simulink model "sim_tvt_2025_pos_ctrl"  (R2020a)
settings: Solver=ode4  StartTime=0.0  StopTime=30.0  FixedStep=0.01  RelTol=1e-3
values from neighbouring files (symbols this model uses):
  alfa = 0.02    [init_tvt_2025_pos_ctrl.m]
  alfa_theta = 20    [init_tvt_2025_pos_ctrl.m]
  alfa_theta_obs = 100    [init_tvt_2025_pos_ctrl.m]
  c0 = 0.1    [init_tvt_2025_pos_ctrl.m]
  c1_diff_sigma_bar_v = diag([25; 30; 20])    [init_tvt_2025_pos_ctrl.m]
  c1v = diag([5.8; 6.5; 6.5])    [init_tvt_2025_pos_ctrl.m]
  c2_diff_sigma_bar_v = diag([50; 50; 10])    [init_tvt_2025_pos_ctrl.m]
  c2v = diag([5.8; 6.5; 6.5])    [init_tvt_2025_pos_ctrl.m]
  c3_diff_sigma_bar_v = diag([15; 15; 10])    [init_tvt_2025_pos_ctrl.m]
  c3v = diag([4.8; 6.4; 6.0])    [init_tvt_2025_pos_ctrl.m]
  delta_p_i_0 = zeros(3, NF)    [init_tvt_2025_pos_ctrl.m]
  delta_v_i_0 = zeros(3, NF)    [init_tvt_2025_pos_ctrl.m]
  dp_aa_t = 0.2 * ones(3, 5) + ( 1.0 - 0.2 ) * rand(3, 5)    [init_tvt_2025_pos_ctrl.m]
  dp_ff_t = [ 0.4 * ones(1, 5) + ( 1.0 - 0.4 ) * rand(1, 5);                      0.4 * ones(1, 5) + ( 1.0 - 0.4 ) * rand(1, 5);                      0.2 * ones(1, 5) + ( 0.6 - 0.2 ) * rand(1, 5) ]    [init_tvt_2025_pos_ctrl.m]
  dp_phi_t = ( - pi / 2 ) * ones(3, 5) + ( pi / 2 - ( - pi / 2 ) ) * rand(3, 5)    [init_tvt_2025_pos_ctrl.m]
  eps0 = [0.05; 0.01; 0.01]    [init_tvt_2025_pos_ctrl.m]
  eta_ld_hat_init = zeros(3,NF)    [init_tvt_2025_pos_ctrl.m]
  etai_0 = zeros(3,5)    [init_tvt_2025_pos_ctrl.m]
  gamma0 = diag([1, 1, 1])    [init_tvt_2025_pos_ctrl.m]
  k_phi = diag([10, 10, 10])    [init_tvt_2025_pos_ctrl.m]
  k_theta = diag([5, 5, 5])    [init_tvt_2025_pos_ctrl.m]
  kai0 = [15; 10; 10]    [init_tvt_2025_pos_ctrl.m]
  kai_1_t = 0.02    [init_tvt_2025_pos_ctrl.m]
  kai_3_t = 0.1    [init_tvt_2025_pos_ctrl.m]
  ksi_ld_hat_init = zeros(3,NF)    [init_tvt_2025_pos_ctrl.m]
  ksii_0 = zeros(3,5)    [init_tvt_2025_pos_ctrl.m]
  l1v = diag([20; 20; 20])    [init_tvt_2025_pos_ctrl.m]
  l2v = diag([30; 30; 30])    [init_tvt_2025_pos_ctrl.m]
  lam0 = [15; 10; 10]    [init_tvt_2025_pos_ctrl.m]
  lam1 = diag([5,5,5])    [init_tvt_2025_pos_ctrl.m]
  lam2 = diag([5,5,5])    [init_tvt_2025_pos_ctrl.m]
  lam3 = diag([5,5,5])    [init_tvt_2025_pos_ctrl.m]
  lam4 = diag([5,5,5])    [init_tvt_2025_pos_ctrl.m]
  Lamd_diff_sigma_bar_v = 0.5    [init_tvt_2025_pos_ctrl.m]
  mass_i = zeros(1,NF)    [init_tvt_2025_pos_ctrl.m]
  Mii = diag([1;0;0;0;1])    [init_tvt_2025_pos_ctrl.m]
  pos0 = zeros(3, 1)    [init_tvt_2025_pos_ctrl.m]
  pos_bar_init = zeros(3,NF)    [init_tvt_2025_pos_ctrl.m]
  PZ0 = P0(3)    [init_tvt_2025_pos_ctrl.m]
  PZ1 = 10    [init_tvt_2025_pos_ctrl.m]
  Qci_init = repmat([1;0;0;0],1,NF)    [init_tvt_2025_pos_ctrl.m]
  R0 = 4    [init_tvt_2025_pos_ctrl.m]
  R1 = 8    [init_tvt_2025_pos_ctrl.m]
  Rx2 = 10    [init_tvt_2025_pos_ctrl.m]
  Ry2 = 6    [init_tvt_2025_pos_ctrl.m]
  Rz2 = 4    [init_tvt_2025_pos_ctrl.m]
  T0 = 0    [init_tvt_2025_pos_ctrl.m]
  T1 = tseq1    (= 10)    [init_tvt_2025_pos_ctrl.m]
  T12 = tseq1 + tseq12    (= 20)    [init_tvt_2025_pos_ctrl.m]
  T2 = tseq1 + tseq12 + tseq2    (= 30)    [init_tvt_2025_pos_ctrl.m]
  theta0 = ( 2 / 5 ) * pi    (= 1.25663706144)    [init_tvt_2025_pos_ctrl.m]
  vel0 = zeros(3, 1)    [init_tvt_2025_pos_ctrl.m]
  vel_bar_init = zeros(3,NF)    [init_tvt_2025_pos_ctrl.m]
  Wij = [0,0,1,0,0;              0,0,1,1,0;              1,0,0,0,1;              0,1,1,0,0;              0,0,1,0,0]    [init_tvt_2025_pos_ctrl.m]
  X1 = 8    [init_tvt_2025_pos_ctrl.m]
  X2 = 2    [init_tvt_2025_pos_ctrl.m]
  X3 = 3    [init_tvt_2025_pos_ctrl.m]
  Y1 = 10    [init_tvt_2025_pos_ctrl.m]
  Y2 = 2    [init_tvt_2025_pos_ctrl.m]
  Y3 = 4    [init_tvt_2025_pos_ctrl.m]
  Z1 = 4    [init_tvt_2025_pos_ctrl.m]
  Z2 = -6    [init_tvt_2025_pos_ctrl.m]
  Z3 = 2    [init_tvt_2025_pos_ctrl.m]
  zeta_diff_sigma_bar_v = 0.08    [init_tvt_2025_pos_ctrl.m]
undefined symbols (not defined in the file or in its folder): cal_frac_squ, p_alfav1, p_alfav2, p_gamma1_pos, p_gamma1_vel, p_gamma2_pos, p_gamma2_vel, q_alfav1, q_alfav2, q_gamma1_pos, q_gamma1_vel, q_gamma2_pos, q_gamma2_vel
(part 3 of 5)

== matlab function sim_tvt_2025_pos_ctrl/cal differentiator d_sigma_bar_v_hat agent 3/cal sig3 ==
  data: x input; z output; y input
function z = fcn(x, y)
z = x(:) .* sign(y(:));

== matlab function sim_tvt_2025_pos_ctrl/cal differentiator d_sigma_bar_v_hat agent 3/cal sig4 ==
  data: x input; z output; y input
function z = fcn(x, y)
z = x(:) .* sign(y(:));

== matlab function sim_tvt_2025_pos_ctrl/cal differentiator d_sigma_bar_v_hat agent 3/cal sig5 ==
  data: x input; z output; y input
function z = fcn(x, y)
z = x(:) .* sign(y(:));

== matlab function sim_tvt_2025_pos_ctrl/cal pos_bar_i agent 1 ==
  data: ksi_i_vec input; phi_vec input; pos_bar_1 output
function pos_bar_1 = fcn(ksi_i_vec, phi_vec)
%%%% 计算辅助位置向量
iiuav = 1;
pos_bar_1 = ksi_i_vec(:,iiuav) - phi_vec(:,iiuav);

== matlab function sim_tvt_2025_pos_ctrl/cal pos_bar_i agent 2 ==
  data: ksi_i_vec input; phi_vec input; pos_bar_2 output
function pos_bar_2 = fcn(ksi_i_vec, phi_vec)
%%%% 计算辅助位置向量
iiuav = 2;
pos_bar_2 = ksi_i_vec(:,iiuav) - phi_vec(:,iiuav);

== matlab function sim_tvt_2025_pos_ctrl/cal differentiator d_sigma_bar_v_hat agent 3/choose sigma_bar_v ==
  data: x input; y output
function y = fcn(x)
iiuav = 3;
y = x(:,iiuav);

== matlab function sim_tvt_2025_pos_ctrl/Phi_sec_sigma_i agent 1 ==
  data: sigma_i_vec input; Phi_sec_sigma_1 output
function Phi_sec_sigma_1 = fcn(sigma_i_vec)
%%%% 跟随者期望速度分布式观测器
iiuav = 1;
Phi_sec_sigma_1 = diag( [ sech( sigma_i_vec(1,iiuav) ) ^ 2, ...
                                                sech( sigma_i_vec(2,iiuav) ) ^ 2, ...
                                                sech( sigma_i_vec(3,iiuav) ) ^ 2 ] );

== matlab function sim_tvt_2025_pos_ctrl/cal differentiator d_sigma_bar_v_hat agent 3/trans to column20 ==
  data: x input; y output
function y = fcn(x)
y = x(:);

== matlab function sim_tvt_2025_pos_ctrl/cal differentiator d_sigma_bar_v_hat agent 3/trans to column21 ==
  data: x input; y output
function y = fcn(x)
y = x(:);

== matlab function sim_tvt_2025_pos_ctrl/cal differentiator d_sigma_bar_v_hat agent 3/trans to column22 ==
  data: x input; y output
function y = fcn(x)
y = x(:);

== matlab function sim_tvt_2025_pos_ctrl/cal differentiator d_sigma_bar_v_hat agent 3/trans to column23 ==
  data: x input; y output
function y = fcn(x)
y = x(:);

== matlab function sim_tvt_2025_pos_ctrl/cal differentiator d_sigma_bar_v_hat agent 3/trans to column24 ==
  data: x input; y output
function y = fcn(x)
y = x(:);

== matlab function sim_tvt_2025_pos_ctrl/cal differentiator d_sigma_bar_v_hat agent 3/trans to column25 ==
  data: x input; y output
function y = fcn(x)
y = x(:);

== matlab function sim_tvt_2025_pos_ctrl/cal differentiator d_sigma_bar_v_hat agent 4/cal differentiator ==
  data: c1 input; d_sigma_bar_v_hat output; d_dsigma_bar_v_hat output; d_d2sigma_bar_v_hat output; c2 input; c3 input; chi_t input; sigma_bar_v_sig_1 input; sigma_bar_v_sig_2 input; sigma_bar_v_sig_3 input; sigma_bar_v_sig_4 input; sigma_bar_v_sig_5 input; sigma_bar_v_sig_6 input; d_sigma_bar_v_hat input; d2_sigma_bar_v_hat input
function [d_sigma_bar_v_hat, d_dsigma_bar_v_hat, d_d2sigma_bar_v_hat] = fcn(c1, c2, c3, chi_t, sigma_bar_v_sig_1, sigma_bar_v_sig_2, sigma_bar_v_sig_3, ...
                                                                                                                                                sigma_bar_v_sig_4, sigma_bar_v_sig_5, sigma_bar_v_sig_6, d_sigma_bar_v_hat, d2_sigma_bar_v_hat)
d_d2sigma_bar_v_hat = -chi_t .* c1 * sigma_bar_v_sig_1(:) - (1 - chi_t) .* c1 * sigma_bar_v_sig_2(:);
d_dsigma_bar_v_hat = -chi_t .* c2 * sigma_bar_v_sig_3(:) - (1 - chi_t) .* c2 * sigma_bar_v_sig_4(:) + d2_sigma_bar_v_hat(:);
d_sigma_bar_v_hat = -chi_t .* c3 * sigma_bar_v_sig_5(:) - (1 - chi_t) .* c3 * sigma_bar_v_sig_6(:) + d_sigma_bar_v_hat(:);

== matlab function sim_tvt_2025_pos_ctrl/cal differentiator d_sigma_bar_v_hat agent 4/cal sig ==
  data: x input; z output; y input
function z = fcn(x, y)
z = x(:) .* sign(y(:));

== matlab function sim_tvt_2025_pos_ctrl/Phi_sec_sigma_i agent 2 ==
  data: sigma_i_vec input; Phi_sec_sigma_2 output
function Phi_sec_sigma_2 = fcn(sigma_i_vec)
%%%% 跟随者期望速度分布式观测器
iiuav = 2;
Phi_sec_sigma_2 = diag( [ sech( sigma_i_vec(1,iiuav) ) ^ 2, ...
                                                sech( sigma_i_vec(2,iiuav) ) ^ 2, ...
                                                sech( sigma_i_vec(3,iiuav) ) ^ 2 ] );

== matlab function sim_tvt_2025_pos_ctrl/cal differentiator d_sigma_bar_v_hat agent 4/cal sig1 ==
  data: x input; z output; y input
function z = fcn(x, y)
z = x(:) .* sign(y(:));

== matlab function sim_tvt_2025_pos_ctrl/cal differentiator d_sigma_bar_v_hat agent 4/cal sig2 ==
  data: x input; z output; y input
function z = fcn(x, y)
z = x(:) .* sign(y(:));

== matlab function sim_tvt_2025_pos_ctrl/cal differentiator d_sigma_bar_v_hat agent 4/cal sig3 ==
  data: x input; z output; y input
function z = fcn(x, y)
z = x(:) .* sign(y(:));

== matlab function sim_tvt_2025_pos_ctrl/cal differentiator d_sigma_bar_v_hat agent 4/cal sig4 ==
  data: x input; z output; y input
function z = fcn(x, y)
z = x(:) .* sign(y(:));

== matlab function sim_tvt_2025_pos_ctrl/cal differentiator d_sigma_bar_v_hat agent 4/cal sig5 ==
  data: x input; z output; y input
function z = fcn(x, y)
z = x(:) .* sign(y(:));

== matlab function sim_tvt_2025_pos_ctrl/cal differentiator d_sigma_bar_v_hat agent 4/choose sigma_bar_v ==
  data: x input; y output
function y = fcn(x)
iiuav = 4;
y = x(:,iiuav);

== matlab function sim_tvt_2025_pos_ctrl/cal differentiator d_sigma_bar_v_hat agent 4/trans to column20 ==
  data: x input; y output
function y = fcn(x)
y = x(:);

== matlab function sim_tvt_2025_pos_ctrl/cal differentiator d_sigma_bar_v_hat agent 4/trans to column21 ==
  data: x input; y output
function y = fcn(x)
y = x(:);

== matlab function sim_tvt_2025_pos_ctrl/cal differentiator d_sigma_bar_v_hat agent 4/trans to column22 ==
  data: x input; y output
function y = fcn(x)
y = x(:);

== matlab function sim_tvt_2025_pos_ctrl/Phi_sec_sigma_i agent 3 ==
  data: sigma_i_vec input; Phi_sec_sigma_3 output
function Phi_sec_sigma_3 = fcn(sigma_i_vec)
%%%% 跟随者期望速度分布式观测器
iiuav = 3;
Phi_sec_sigma_3 = diag( [ sech( sigma_i_vec(1,iiuav) ) ^ 2, ...
                                                sech( sigma_i_vec(2,iiuav) ) ^ 2, ...
                                                sech( sigma_i_vec(3,iiuav) ) ^ 2 ] );

== matlab function sim_tvt_2025_pos_ctrl/cal differentiator d_sigma_bar_v_hat agent 4/trans to column23 ==
  data: x input; y output
function y = fcn(x)
y = x(:);

== matlab function sim_tvt_2025_pos_ctrl/cal Rci from ui ==
  data: Rci output; mi_vec input; ui_vec input
function Rci = fcn(mi_vec, ui_vec)
Rci = zeros(3,3,5);
for iiuav = 1:5
    Rci(:,:,iiuav) = cal_Rc_with_u(mi_vec(iiuav), ui_vec(:,iiuav));
end

end

== matlab function sim_tvt_2025_pos_ctrl/cal differentiator d_sigma_bar_v_hat agent 4/trans to column24 ==
  data: x input; y output
function y = fcn(x)
y = x(:);

== matlab function sim_tvt_2025_pos_ctrl/cal differentiator d_sigma_bar_v_hat agent 4/trans to column25 ==
  data: x input; y output
function y = fcn(x)
y = x(:);

== matlab function sim_tvt_2025_pos_ctrl/cal differentiator d_sigma_bar_v_hat agent 5/cal differentiator ==
  data: c1 input; d_sigma_bar_v_hat output; d_dsigma_bar_v_hat output; d_d2sigma_bar_v_hat output; c2 input; c3 input; chi_t input; sigma_bar_v_sig_1 input; sigma_bar_v_sig_2 input; sigma_bar_v_sig_3 input; sigma_bar_v_sig_4 input; sigma_bar_v_sig_5 input; sigma_bar_v_sig_6 input; d_sigma_bar_v_hat input; d2_sigma_bar_v_hat input
function [d_sigma_bar_v_hat, d_dsigma_bar_v_hat, d_d2sigma_bar_v_hat] = fcn(c1, c2, c3, chi_t, sigma_bar_v_sig_1, sigma_bar_v_sig_2, sigma_bar_v_sig_3, ...
                                                                                                                                                sigma_bar_v_sig_4, sigma_bar_v_sig_5, sigma_bar_v_sig_6, d_sigma_bar_v_hat, d2_sigma_bar_v_hat)
d_d2sigma_bar_v_hat = -chi_t .* c1 * sigma_bar_v_sig_1(:) - (1 - chi_t) .* c1 * sigma_bar_v_sig_2(:);
d_dsigma_bar_v_hat = -chi_t .* c2 * sigma_bar_v_sig_3(:) - (1 - chi_t) .* c2 * sigma_bar_v_sig_4(:) + d2_sigma_bar_v_hat(:);
d_sigma_bar_v_hat = -chi_t .* c3 * sigma_bar_v_sig_5(:) - (1 - chi_t) .* c3 * sigma_bar_v_sig_6(:) + d_sigma_bar_v_hat(:);

== matlab function sim_tvt_2025_pos_ctrl/cal differentiator d_sigma_bar_v_hat agent 5/cal sig ==
  data: x input; z output; y input
function z = fcn(x, y)
z = x(:) .* sign(y(:));

== matlab function sim_tvt_2025_pos_ctrl/cal differentiator d_sigma_bar_v_hat agent 5/cal sig1 ==
  data: x input; z output; y input
function z = fcn(x, y)
z = x(:) .* sign(y(:));

== matlab function sim_tvt_2025_pos_ctrl/cal differentiator d_sigma_bar_v_hat agent 5/cal sig2 ==
  data: x input; z output; y input
function z = fcn(x, y)
z = x(:) .* sign(y(:));

== matlab function sim_tvt_2025_pos_ctrl/Phi_sec_sigma_i agent 4 ==
  data: sigma_i_vec input; Phi_sec_sigma_4 output
function Phi_sec_sigma_4 = fcn(sigma_i_vec)
%%%% 跟随者期望速度分布式观测器
iiuav = 4;
Phi_sec_sigma_4 = diag( [ sech( sigma_i_vec(1,iiuav) ) ^ 2, ...
                                                sech( sigma_i_vec(2,iiuav) ) ^ 2, ...
                                                sech( sigma_i_vec(3,iiuav) ) ^ 2 ] );

== matlab function sim_tvt_2025_pos_ctrl/cal differentiator d_sigma_bar_v_hat agent 5/cal sig3 ==
  data: x input; z output; y input
function z = fcn(x, y)
z = x(:) .* sign(y(:));

== matlab function sim_tvt_2025_pos_ctrl/cal differentiator d_sigma_bar_v_hat agent 5/cal sig4 ==
  data: x input; z output; y input
function z = fcn(x, y)
z = x(:) .* sign(y(:));

== matlab function sim_tvt_2025_pos_ctrl/cal differentiator d_sigma_bar_v_hat agent 5/cal sig5 ==
  data: x input; z output; y input
function z = fcn(x, y)
z = x(:) .* sign(y(:));

== matlab function sim_tvt_2025_pos_ctrl/cal differentiator d_sigma_bar_v_hat agent 5/choose sigma_bar_v ==
  data: x input; y output
function y = fcn(x)
iiuav = 5;
y = x(:,iiuav);

== matlab function sim_tvt_2025_pos_ctrl/cal differentiator d_sigma_bar_v_hat agent 5/trans to column20 ==
  data: x input; y output
function y = fcn(x)
y = x(:);

== matlab function sim_tvt_2025_pos_ctrl/cal differentiator d_sigma_bar_v_hat agent 5/trans to column21 ==
  data: x input; y output
function y = fcn(x)
y = x(:);

== matlab function sim_tvt_2025_pos_ctrl/cal differentiator d_sigma_bar_v_hat agent 5/trans to column22 ==
  data: x input; y output
function y = fcn(x)
y = x(:);

== matlab function sim_tvt_2025_pos_ctrl/cal differentiator d_sigma_bar_v_hat agent 5/trans to column23 ==
  data: x input; y output
function y = fcn(x)
y = x(:);

== matlab function sim_tvt_2025_pos_ctrl/cal differentiator d_sigma_bar_v_hat agent 5/trans to column24 ==
  data: x input; y output
function y = fcn(x)
y = x(:);

== matlab function sim_tvt_2025_pos_ctrl/Phi_sec_sigma_i agent 5 ==
  data: sigma_i_vec input; Phi_sec_sigma_5 output
function Phi_sec_sigma_5 = fcn(sigma_i_vec)
%%%% 跟随者期望速度分布式观测器
iiuav = 5;
Phi_sec_sigma_5 = diag( [ sech( sigma_i_vec(1,iiuav) ) ^ 2, ...
                                                sech( sigma_i_vec(2,iiuav) ) ^ 2, ...
                                                sech( sigma_i_vec(3,iiuav) ) ^ 2 ] );

== matlab function sim_tvt_2025_pos_ctrl/cal differentiator d_sigma_bar_v_hat agent 5/trans to column25 ==
  data: x input; y output
function y = fcn(x)
y = x(:);

== matlab function sim_tvt_2025_pos_ctrl/combine d_sigma_bar_v_est ==
  data: d_sigma_bar_v_est_1 input; d_sigma_bar_v_est_2 input; d_sigma_bar_v_est_3 input; d_sigma_bar_v_est_4 input; d_sigma_bar_v_est_5 input; d_sigma_bar_v_vec output
function d_sigma_bar_v_vec  = fcn(d_sigma_bar_v_est_1, d_sigma_bar_v_est_2, d_sigma_bar_v_est_3, d_sigma_bar_v_est_4, d_sigma_bar_v_est_5)
%%%% 合并用微分器求得的虚拟速度控制量导数
d_sigma_bar_v_vec = [d_sigma_bar_v_est_1(:), d_sigma_bar_v_est_2(:), d_sigma_bar_v_est_3(:), d_sigma_bar_v_est_4(:), d_sigma_bar_v_est_5(:)];

== matlab function sim_tvt_2025_pos_ctrl/cal abs 21 ==
  data: x input; y output
function y = fcn(x)
y = abs(x(:));

== matlab function sim_tvt_2025_pos_ctrl/cal abs 22 ==
  data: x input; y output
function y = fcn(x)
y = abs(x(:));

== matlab function sim_tvt_2025_pos_ctrl/choose ksi_est_err 21 ==
  data: x input; y output
function y = fcn(x)
iiuav = 1;
y = x(:,iiuav);

== matlab function sim_tvt_2025_pos_ctrl/choose ksi_est_err 22 ==
  data: x input; y output
function y = fcn(x)
iiuav = 1;
y = x(:,iiuav);

== matlab function sim_tvt_2025_pos_ctrl/trans to column20 ==
  data: x input; y output
function y = fcn(x)
y = x(:);

== matlab function sim_tvt_2025_pos_ctrl/trans to column21 ==
  data: x input; y output
function y = fcn(x)
y = x(:);

== matlab function sim_tvt_2025_pos_ctrl/cal theta_sigma_bar_v_tilt agent 1 ==
  data: alfa_theta input; sigma_bar_v_tilt_squ_1_1 input; theta_sigma_bar_v_tilt_1_1 output; sigma_bar_v_tilt_squ_2_1 input; sigma_bar_v_tilt_vec input; theta_sigma_bar_v_tilt_2_1 output
function [theta_sigma_bar_v_tilt_1_1, theta_sigma_bar_v_tilt_2_1] = fcn(alfa_theta, sigma_bar_v_tilt_squ_1_1, sigma_bar_v_tilt_squ_2_1, sigma_bar_v_tilt_vec)
%%%% 计算平滑递增函数
iiuav = 1;
theta_sigma_bar_v_tilt_1_1 = sigma_bar_v_tilt_squ_1_1(:) .* ( -1 + 2 ./ ( 1 + exp( -alfa_theta .* sigma_bar_v_tilt_vec(:,iiuav) ) ) );
theta_sigma_bar_v_tilt_2_1 = sigma_bar_v_tilt_squ_2_1(:) .* ( -1 + 2 ./ ( 1 + exp( -alfa_theta .* sigma_bar_v_tilt_vec(:,iiuav) ) ) );

== matlab function sim_tvt_2025_pos_ctrl/combine beta_hat ==
  data: beta_hat_1 input; beta_hat_vec output; beta_hat_2 input; beta_hat_3 input; beta_hat_4 input; beta_hat_5 input
function beta_hat_vec  = fcn(beta_hat_1, beta_hat_2, beta_hat_3, beta_hat_4, beta_hat_5)
%%%% 合并自适应律
beta_hat_vec = [beta_hat_1, beta_hat_2, beta_hat_3, beta_hat_4, beta_hat_5];

== matlab function sim_tvt_2025_pos_ctrl/cal abs 23 ==
  data: x input; y output
function y = fcn(x)
y = abs(x(:));

== matlab function sim_tvt_2025_pos_ctrl/cal abs 24 ==
  data: x input; y output
function y = fcn(x)
y = abs(x(:));

== matlab function sim_tvt_2025_pos_ctrl/cal theta_sigma_bar_v_tilt agent 2 ==
  data: alfa_theta input; sigma_bar_v_tilt_squ_1_2 input; theta_sigma_bar_v_tilt_1_2 output; sigma_bar_v_tilt_squ_2_2 input; sigma_bar_v_tilt_vec input; theta_sigma_bar_v_tilt_2_2 output
function [theta_sigma_bar_v_tilt_1_2, theta_sigma_bar_v_tilt_2_2] = fcn(alfa_theta, sigma_bar_v_tilt_squ_1_2, sigma_bar_v_tilt_squ_2_2, sigma_bar_v_tilt_vec)
%%%% 计算平滑递增函数
iiuav = 2;
theta_sigma_bar_v_tilt_1_2 = sigma_bar_v_tilt_squ_1_2(:) .* ( -1 + 2 ./ ( 1 + exp( -alfa_theta .* sigma_bar_v_tilt_vec(:,iiuav) ) ) );
theta_sigma_bar_v_tilt_2_2 = sigma_bar_v_tilt_squ_2_2(:) .* ( -1 + 2 ./ ( 1 + exp( -alfa_theta .* sigma_bar_v_tilt_vec(:,iiuav) ) ) );

== matlab function sim_tvt_2025_pos_ctrl/choose ksi_est_err 23 ==
  data: x input; y output
function y = fcn(x)
iiuav = 2;
y = x(:,iiuav);

== matlab function sim_tvt_2025_pos_ctrl/choose ksi_est_err 24 ==
  data: x input; y output
function y = fcn(x)
iiuav = 2;
y = x(:,iiuav);

== matlab function sim_tvt_2025_pos_ctrl/trans to column22 ==
  data: x input; y output
function y = fcn(x)
y = x(:);

== matlab function sim_tvt_2025_pos_ctrl/trans to column23 ==
  data: x input; y output
function y = fcn(x)
y = x(:);

== matlab function sim_tvt_2025_pos_ctrl/cal abs 25 ==
  data: x input; y output
function y = fcn(x)
y = abs(x(:));

== matlab function sim_tvt_2025_pos_ctrl/cal abs 26 ==
  data: x input; y output
function y = fcn(x)
y = abs(x(:));

== matlab function sim_tvt_2025_pos_ctrl/cal theta_sigma_bar_v_tilt agent 3 ==
  data: alfa_theta input; sigma_bar_v_tilt_squ_1_3 input; theta_sigma_bar_v_tilt_1_3 output; sigma_bar_v_tilt_squ_2_3 input; sigma_bar_v_tilt_vec input; theta_sigma_bar_v_tilt_2_3 output
function [theta_sigma_bar_v_tilt_1_3, theta_sigma_bar_v_tilt_2_3] = fcn(alfa_theta, sigma_bar_v_tilt_squ_1_3, sigma_bar_v_tilt_squ_2_3, sigma_bar_v_tilt_vec)
%%%% 计算平滑递增函数
iiuav = 3;
theta_sigma_bar_v_tilt_1_3 = sigma_bar_v_tilt_squ_1_3(:) .* ( -1 + 2 ./ ( 1 + exp( -alfa_theta .* sigma_bar_v_tilt_vec(:,iiuav) ) ) );
theta_sigma_bar_v_tilt_2_3 = sigma_bar_v_tilt_squ_2_3(:) .* ( -1 + 2 ./ ( 1 + exp( -alfa_theta .* sigma_bar_v_tilt_vec(:,iiuav) ) ) );

== matlab function sim_tvt_2025_pos_ctrl/choose ksi_est_err 25 ==
  data: x input; y output
function y = fcn(x)
iiuav = 3;
y = x(:,iiuav);

== matlab function sim_tvt_2025_pos_ctrl/choose ksi_est_err 26 ==
  data: x input; y output
function y = fcn(x)
iiuav = 3;
y = x(:,iiuav);

== matlab function sim_tvt_2025_pos_ctrl/trans to column24 ==
  data: x input; y output
function y = fcn(x)
y = x(:);

== matlab function sim_tvt_2025_pos_ctrl/trans to column25 ==
  data: x input; y output
function y = fcn(x)
y = x(:);

== matlab function sim_tvt_2025_pos_ctrl/cal abs 27 ==
  data: x input; y output
function y = fcn(x)
y = abs(x(:));

== matlab function sim_tvt_2025_pos_ctrl/update betai agent 1 ==
  data: eps0 input; d_beta_hat_1 output; Wij input; Mii input; tsim input; u0 input; rho_hat_vec input
function d_beta_hat_1 = fcn(eps0, Wij, Mii, tsim, u0, rho_hat_vec)
%%%% 自适应律
iiuav = 1;
err_rho = Mii(iiuav, iiuav) * ( rho_hat_vec(:,iiuav) - u0(:) );
for jjuav = 1:5
    err_rho = err_rho + Wij(iiuav, jjuav) * ( rho_hat_vec(:,iiuav) - rho_hat_vec(:,jjuav) );
end
d_beta_hat_1 = ( err_rho(:)' ) * tanh( err_rho(:) ./ exp( -eps0 * tsim ) );

== matlab function sim_tvt_2025_pos_ctrl/cal abs 28 ==
  data: x input; y output
function y = fcn(x)
y = abs(x(:));

== matlab function sim_tvt_2025_pos_ctrl/cal theta_sigma_bar_v_tilt agent 4 ==
  data: alfa_theta input; sigma_bar_v_tilt_squ_1_4 input; theta_sigma_bar_v_tilt_1_4 output; sigma_bar_v_tilt_squ_2_4 input; sigma_bar_v_tilt_vec input; theta_sigma_bar_v_tilt_2_4 output
function [theta_sigma_bar_v_tilt_1_4, theta_sigma_bar_v_tilt_2_4] = fcn(alfa_theta, sigma_bar_v_tilt_squ_1_4, sigma_bar_v_tilt_squ_2_4, sigma_bar_v_tilt_vec)
%%%% 计算平滑递增函数
iiuav = 4;
theta_sigma_bar_v_tilt_1_4 = sigma_bar_v_tilt_squ_1_4(:) .* ( -1 + 2 ./ ( 1 + exp( -alfa_theta .* sigma_bar_v_tilt_vec(:,iiuav) ) ) );
theta_sigma_bar_v_tilt_2_4 = sigma_bar_v_tilt_squ_2_4(:) .* ( -1 + 2 ./ ( 1 + exp( -alfa_theta .* sigma_bar_v_tilt_vec(:,iiuav) ) ) );

== matlab function sim_tvt_2025_pos_ctrl/choose ksi_est_err 27 ==
  data: x input; y output
function y = fcn(x)
iiuav = 4;
y = x(:,iiuav);

== matlab function sim_tvt_2025_pos_ctrl/choose ksi_est_err 28 ==
  data: x input; y output
function y = fcn(x)
iiuav = 4;
y = x(:,iiuav);

== matlab function sim_tvt_2025_pos_ctrl/trans to column26 ==
  data: x input; y output
function y = fcn(x)
y = x(:);

== matlab function sim_tvt_2025_pos_ctrl/trans to column27 ==
  data: x input; y output
function y = fcn(x)
y = x(:);

== matlab function sim_tvt_2025_pos_ctrl/cal abs 29 ==
  data: x input; y output
function y = fcn(x)
y = abs(x(:));

== matlab function sim_tvt_2025_pos_ctrl/cal abs 30 ==
  data: x input; y output
function y = fcn(x)
y = abs(x(:));

== matlab function sim_tvt_2025_pos_ctrl/cal theta_sigma_bar_v_tilt agent 5 ==
  data: alfa_theta input; sigma_bar_v_tilt_squ_1_5 input; theta_sigma_bar_v_tilt_1_5 output; sigma_bar_v_tilt_squ_2_5 input; sigma_bar_v_tilt_vec input; theta_sigma_bar_v_tilt_2_5 output
function [theta_sigma_bar_v_tilt_1_5, theta_sigma_bar_v_tilt_2_5] = fcn(alfa_theta, sigma_bar_v_tilt_squ_1_5, sigma_bar_v_tilt_squ_2_5, sigma_bar_v_tilt_vec)
%%%% 计算平滑递增函数
iiuav = 5;
theta_sigma_bar_v_tilt_1_5 = sigma_bar_v_tilt_squ_1_5(:) .* ( -1 + 2 ./ ( 1 + exp( -alfa_theta .* sigma_bar_v_tilt_vec(:,iiuav) ) ) );
theta_sigma_bar_v_tilt_2_5 = sigma_bar_v_tilt_squ_2_5(:) .* ( -1 + 2 ./ ( 1 + exp( -alfa_theta .* sigma_bar_v_tilt_vec(:,iiuav) ) ) );

== matlab function sim_tvt_2025_pos_ctrl/choose ksi_est_err 29 ==
  data: x input; y output
function y = fcn(x)
iiuav = 5;
y = x(:,iiuav);

== matlab function sim_tvt_2025_pos_ctrl/choose ksi_est_err 30 ==
  data: x input; y output
function y = fcn(x)
iiuav = 5;
y = x(:,iiuav);

== matlab function sim_tvt_2025_pos_ctrl/trans to column28 ==
  data: x input; y output
function y = fcn(x)
y = x(:);

== matlab function sim_tvt_2025_pos_ctrl/trans to column29 ==
  data: x input; y output
function y = fcn(x)
y = x(:);

== matlab function sim_tvt_2025_pos_ctrl/combine theta_sigma_bar_v_tilt ==
  data: theta_sigma_bar_v_tilt_1_1 input; theta_sigma_bar_v_tilt_1_2 input; theta_sigma_bar_v_tilt_1_3 input; theta_sigma_bar_v_tilt_1_4 input; theta_sigma_bar_v_tilt_1_5 input; theta_sigma_bar_v_tilt_1_vec output; theta_sigma_bar_v_tilt_2_1 input; theta_sigma_bar_v_tilt_2_vec output; theta_sigma_bar_v_tilt_2_2 input; theta_sigma_bar_v_tilt_2_3 input; theta_sigma_bar_v_tilt_2_4 input; theta_sigma_bar_v_tilt_2_5 input
function [theta_sigma_bar_v_tilt_1_vec, theta_sigma_bar_v_tilt_2_vec]  = fcn(theta_sigma_bar_v_tilt_1_1, theta_sigma_bar_v_tilt_1_2, theta_sigma_bar_v_tilt_1_3, theta_sigma_bar_v_tilt_1_4, theta_sigma_bar_v_tilt_1_5, ...
                                                                                                                                            theta_sigma_bar_v_tilt_2_1, theta_sigma_bar_v_tilt_2_2, theta_sigma_bar_v_tilt_2_3, theta_sigma_bar_v_tilt_2_4, theta_sigma_bar_v_tilt_2_5)
%%%% 合并领导者位置观测器输出结果
theta_sigma_bar_v_tilt_1_vec = [theta_sigma_bar_v_tilt_1_1(:), theta_sigma_bar_v_tilt_1_2(:), theta_sigma_bar_v_tilt_1_3(:), theta_sigma_bar_v_tilt_1_4(:), theta_sigma_bar_v_tilt_1_5(:)];
theta_sigma_bar_v_tilt_2_vec = [theta_sigma_bar_v_tilt_2_1(:), theta_sigma_bar_v_tilt_2_2(:), theta_sigma_bar_v_tilt_2_3(:), theta_sigma_bar_v_tilt_2_4(:), theta_sigma_bar_v_tilt_2_5(:)];

== matlab function sim_tvt_2025_pos_ctrl/update betai agent 2 ==
  data: eps0 input; d_beta_hat_2 output; Wij input; Mii input; tsim input; u0 input; rho_hat_vec input
function d_beta_hat_2 = fcn(eps0, Wij, Mii, tsim, u0, rho_hat_vec)
%%%% 自适应律
iiuav = 2;
err_rho = Mii(iiuav, iiuav) * ( rho_hat_vec(:,iiuav) - u0(:) );
for jjuav = 1:5
    err_rho = err_rho + Wij(iiuav, jjuav) * ( rho_hat_vec(:,iiuav) - rho_hat_vec(:,jjuav) );
end
d_beta_hat_2 = ( err_rho(:)' ) * tanh( err_rho(:) ./ exp( -eps0 * tsim ) );

== matlab function sim_tvt_2025_pos_ctrl/cal sigma_bar_v_hat agent 1 ==
  data: c1v input; c2v input; theta_sigma_bar_v_tilt_1_vec input; d_sigma_bar_v_hat_1 output; theta_sigma_bar_v_tilt_2_vec input; d_sigma_bar_v_vec input
function d_sigma_bar_v_hat_1 = fcn(c1v, c2v, theta_sigma_bar_v_tilt_1_vec, theta_sigma_bar_v_tilt_2_vec, d_sigma_bar_v_vec)
%%%% 计算扰动观测器中虚拟速度控制量观测值sigma_v_hat的微分方程
iiuav = 1;
d_sigma_bar_v_hat_1 = d_sigma_bar_v_vec(:,iiuav) + ...
                                            c1v * theta_sigma_bar_v_tilt_1_vec(:,iiuav) + ...
                                            c2v * theta_sigma_bar_v_tilt_2_vec(:,iiuav);

== matlab function sim_tvt_2025_pos_ctrl/cal sigma_bar_v_hat agent 2 ==
  data: c1v input; c2v input; theta_sigma_bar_v_tilt_1_vec input; d_sigma_bar_v_hat_2 output; theta_sigma_bar_v_tilt_2_vec input; d_sigma_bar_v_vec input
function d_sigma_bar_v_hat_2 = fcn(c1v, c2v, theta_sigma_bar_v_tilt_1_vec, theta_sigma_bar_v_tilt_2_vec, d_sigma_bar_v_vec)
%%%% 计算扰动观测器中虚拟速度控制量观测值sigma_v_hat的微分方程
iiuav = 2;
d_sigma_bar_v_hat_2 = d_sigma_bar_v_vec(:,iiuav) + ...
                                            c1v * theta_sigma_bar_v_tilt_1_vec(:,iiuav) + ...
                                            c2v * theta_sigma_bar_v_tilt_2_vec(:,iiuav);

== matlab function sim_tvt_2025_pos_ctrl/cal sigma_bar_v_hat agent 3 ==
  data: c1v input; c2v input; theta_sigma_bar_v_tilt_1_vec input; d_sigma_bar_v_hat_3 output; theta_sigma_bar_v_tilt_2_vec input; d_sigma_bar_v_vec input
function d_sigma_bar_v_hat_3 = fcn(c1v, c2v, theta_sigma_bar_v_tilt_1_vec, theta_sigma_bar_v_tilt_2_vec, d_sigma_bar_v_vec)
%%%% 计算扰动观测器中虚拟速度控制量观测值sigma_v_hat的微分方程
iiuav = 3;
d_sigma_bar_v_hat_3 = d_sigma_bar_v_vec(:,iiuav) + ...
                                            c1v * theta_sigma_bar_v_tilt_1_vec(:,iiuav) + ...
                                            c2v * theta_sigma_bar_v_tilt_2_vec(:,iiuav);

== matlab function sim_tvt_2025_pos_ctrl/cal sigma_bar_v_hat agent 4 ==
  data: c1v input; c2v input; theta_sigma_bar_v_tilt_1_vec input; d_sigma_bar_v_hat_4 output; theta_sigma_bar_v_tilt_2_vec input; d_sigma_bar_v_vec input
function d_sigma_bar_v_hat_4 = fcn(c1v, c2v, theta_sigma_bar_v_tilt_1_vec, theta_sigma_bar_v_tilt_2_vec, d_sigma_bar_v_vec)
%%%% 计算扰动观测器中虚拟速度控制量观测值sigma_v_hat的微分方程
iiuav = 4;
d_sigma_bar_v_hat_4 = d_sigma_bar_v_vec(:,iiuav) + ...
                                            c1v * theta_sigma_bar_v_tilt_1_vec(:,iiuav) + ...
                                            c2v * theta_sigma_bar_v_tilt_2_vec(:,iiuav);

== matlab function sim_tvt_2025_pos_ctrl/cal sigma_bar_v_hat agent 5 ==
  data: c1v input; c2v input; theta_sigma_bar_v_tilt_1_vec input; d_sigma_bar_v_hat_5 output; theta_sigma_bar_v_tilt_2_vec input; d_sigma_bar_v_vec input
function d_sigma_bar_v_hat_5 = fcn(c1v, c2v, theta_sigma_bar_v_tilt_1_vec, theta_sigma_bar_v_tilt_2_vec, d_sigma_bar_v_vec)
%%%% 计算扰动观测器中虚拟速度控制量观测值sigma_v_hat的微分方程
iiuav = 5;
d_sigma_bar_v_hat_5 = d_sigma_bar_v_vec(:,iiuav) + ...
                                            c1v * theta_sigma_bar_v_tilt_1_vec(:,iiuav) + ...
                                            c2v * theta_sigma_bar_v_tilt_2_vec(:,iiuav);

== matlab function sim_tvt_2025_pos_ctrl/cal combine sigma_bar_v_tilt ==
  data: sigma_bar_v_vec input; sigma_bar_v_hat_vec input; sigma_bar_v_tilt_vec output
function sigma_bar_v_tilt_vec = fcn(sigma_bar_v_vec, sigma_bar_v_hat_vec)
%%%% 计算虚拟速度观测误差sigma_bar_v_tilt
sigma_bar_v_tilt_vec = zeros(3,5);
for iiuav = 1:5
    sigma_bar_v_tilt_vec(:,iiuav) = sigma_bar_v_vec(:,iiuav) - sigma_bar_v_hat_vec(:,iiuav);
end

== matlab function sim_tvt_2025_pos_ctrl/combine sigma_bar_v_hat ==
  data: sigma_bar_v_hat_1 input; sigma_bar_v_hat_2 input; sigma_bar_v_hat_3 input; sigma_bar_v_hat_4 input; sigma_bar_v_hat_5 input; sigma_bar_v_hat_vec output
function sigma_bar_v_hat_vec  = fcn(sigma_bar_v_hat_1, sigma_bar_v_hat_2, sigma_bar_v_hat_3, sigma_bar_v_hat_4, sigma_bar_v_hat_5)
%%%% 合并虚拟速度控制量观测值sigma_bar_v_hat
sigma_bar_v_hat_vec = [sigma_bar_v_hat_1(:), sigma_bar_v_hat_2(:), sigma_bar_v_hat_3(:), sigma_bar_v_hat_4(:), sigma_bar_v_hat_5(:)];

== matlab function sim_tvt_2025_pos_ctrl/cal dp_hat agent 1 ==
  data: c3v input; d_sigma_bar_v_vec input; sigma_bar_v_hat_vec input; dp_hat_1 output
function dp_hat_1 = fcn(c3v, d_sigma_bar_v_vec, sigma_bar_v_hat_vec)
%%%% 计算扰动观测值dp_hat
iiuav = 1;
dp_hat_1 = d_sigma_bar_v_vec(:,iiuav) + c3v * sigma_bar_v_hat_vec(:,iiuav);

== matlab function sim_tvt_2025_pos_ctrl/cal dp_hat agent 2 ==
  data: c3v input; d_sigma_bar_v_vec input; sigma_bar_v_hat_vec input; dp_hat_2 output
function dp_hat_2 = fcn(c3v, d_sigma_bar_v_vec, sigma_bar_v_hat_vec)
%%%% 计算扰动观测值dp_hat
iiuav = 2;
dp_hat_2 = d_sigma_bar_v_vec(:,iiuav) + c3v * sigma_bar_v_hat_vec(:,iiuav);

== matlab function sim_tvt_2025_pos_ctrl/cal dp_hat agent 3 ==
  data: c3v input; d_sigma_bar_v_vec input; sigma_bar_v_hat_vec input; dp_hat_3 output
function dp_hat_3 = fcn(c3v, d_sigma_bar_v_vec, sigma_bar_v_hat_vec)
%%%% 计算扰动观测值dp_hat
iiuav = 3;
dp_hat_3 = d_sigma_bar_v_vec(:,iiuav) + c3v * sigma_bar_v_hat_vec(:,iiuav);

== matlab function sim_tvt_2025_pos_ctrl/cal dp_hat agent 4 ==
  data: c3v input; d_sigma_bar_v_vec input; sigma_bar_v_hat_vec input; dp_hat_4 output
function dp_hat_4 = fcn(c3v, d_sigma_bar_v_vec, sigma_bar_v_hat_vec)
%%%% 计算扰动观测值dp_hat
iiuav = 4;
dp_hat_4 = d_sigma_bar_v_vec(:,iiuav) + c3v * sigma_bar_v_hat_vec(:,iiuav);

== matlab function sim_tvt_2025_pos_ctrl/cal dp_hat agent 5 ==
  data: c3v input; d_sigma_bar_v_vec input; sigma_bar_v_hat_vec input; dp_hat_5 output
function dp_hat_5 = fcn(c3v, d_sigma_bar_v_vec, sigma_bar_v_hat_vec)
%%%% 计算扰动观测值dp_hat
iiuav = 5;
dp_hat_5 = d_sigma_bar_v_vec(:,iiuav) + c3v * sigma_bar_v_hat_vec(:,iiuav);

== matlab function sim_tvt_2025_pos_ctrl/update betai agent 3 ==
  data: eps0 input; d_beta_hat_3 output; Wij input; Mii input; tsim input; u0 input; rho_hat_vec input
function d_beta_hat_3 = fcn(eps0, Wij, Mii, tsim, u0, rho_hat_vec)
%%%% 自适应律
iiuav = 3;
err_rho = Mii(iiuav, iiuav) * ( rho_hat_vec(:,iiuav) - u0(:) );
for jjuav = 1:5
    err_rho = err_rho + Wij(iiuav, jjuav) * ( rho_hat_vec(:,iiuav) - rho_hat_vec(:,jjuav) );
end
d_beta_hat_3 = ( err_rho(:)' ) * tanh( err_rho(:) ./ exp( -eps0 * tsim ) );

== matlab function sim_tvt_2025_pos_ctrl/combine dp_hat ==
  data: dp_hat_1 input; dp_hat_2 input; dp_hat_3 input; dp_hat_4 input; dp_hat_5 input; dp_hat_vec output
function dp_hat_vec  = fcn(dp_hat_1, dp_hat_2, dp_hat_3, dp_hat_4, dp_hat_5)
%%%% 合并扰动观测值dp_hat
dp_hat_vec = [dp_hat_1(:), dp_hat_2(:), dp_hat_3(:), dp_hat_4(:), dp_hat_5(:)];

== matlab function sim_tvt_2025_pos_ctrl/cal pos_bar_i agent 3 ==
  data: ksi_i_vec input; phi_vec input; pos_bar_3 output
function pos_bar_3 = fcn(ksi_i_vec, phi_vec)
%%%% 计算辅助位置向量
iiuav = 3;
pos_bar_3 = ksi_i_vec(:,iiuav) - phi_vec(:,iiuav);

== matlab function sim_tvt_2025_pos_ctrl/cal pos_bar_i agent 4 ==
  data: ksi_i_vec input; phi_vec input; pos_bar_4 output
function pos_bar_4 = fcn(ksi_i_vec, phi_vec)
%%%% 计算辅助位置向量
iiuav = 4;
pos_bar_4 = ksi_i_vec(:,iiuav) - phi_vec(:,iiuav);

== matlab function sim_tvt_2025_pos_ctrl/cal pos_bar_i agent 5 ==
  data: ksi_i_vec input; phi_vec input; pos_bar_5 output
function pos_bar_5 = fcn(ksi_i_vec, phi_vec)
%%%% 计算辅助位置向量
iiuav = 5;
pos_bar_5 = ksi_i_vec(:,iiuav) - phi_vec(:,iiuav);

== matlab function sim_tvt_2025_pos_ctrl/combine pos_bar_i ==
  data: pos_bar_1 input; pos_bar_vec output; pos_bar_2 input; pos_bar_3 input; pos_bar_4 input; pos_bar_5 input
function pos_bar_vec  = fcn(pos_bar_1, pos_bar_2, pos_bar_3, pos_bar_4, pos_bar_5)
%%%% 合并辅助位置向量
pos_bar_vec = zeros(3,5);
pos_bar_vec(:,1) = pos_bar_1(:);
pos_bar_vec(:,2) = pos_bar_2(:);
pos_bar_vec(:,3) = pos_bar_3(:);
pos_bar_vec(:,4) = pos_bar_4(:);
pos_bar_vec(:,5) = pos_bar_5(:);

== matlab function sim_tvt_2025_pos_ctrl/update event trigger state agent 1 ==
  data: tk_1 output; c0 input; alfa input; tsim input; pos_bar_vec input; ksi_ld_hat_vec input; tk_vec input; pos_bar_tk_vec input; pos_bar_tk_1 output; ksi_ld_hat_tk_1 output; ksi_ld_hat_tk_vec input
function [tk_1, pos_bar_tk_1, ksi_ld_hat_tk_1] = fcn(c0, alfa, tsim, pos_bar_vec, ksi_ld_hat_vec, tk_vec, pos_bar_tk_vec, ksi_ld_hat_tk_vec)
%%%% 更新事件触发时刻以及对应的状态反馈
iiuav = 1;
err_trig = pos_bar_vec(:,iiuav) - pos_bar_tk_vec(:,iiuav) - ( ksi_ld_hat_vec(:,iiuav) - ksi_ld_hat_tk_vec(:,iiuav) );
err_trig_norm = norm( err_trig(:), 2 );
err_trig_threshold = c0 * exp( -alfa * tsim );
if err_trig_norm >= err_trig_threshold
    tk_1 = tsim;
    pos_bar_tk_1 = pos_bar_vec(:,iiuav);
    ksi_ld_hat_tk_1 = ksi_ld_hat_vec(:,iiuav);
else
    tk_1 = tk_vec(iiuav);
    pos_bar_tk_1 = pos_bar_tk_vec(:,iiuav);
    ksi_ld_hat_tk_1 = ksi_ld_hat_tk_vec(:,iiuav);
end

== matlab function sim_tvt_2025_pos_ctrl/update event trigger state agent 2 ==
  data: tk_2 output; c0 input; alfa input; tsim input; pos_bar_vec input; ksi_ld_hat_vec input; tk_vec input; pos_bar_tk_vec input; pos_bar_tk_2 output; ksi_ld_hat_tk_2 output; ksi_ld_hat_tk_vec input
function [tk_2, pos_bar_tk_2, ksi_ld_hat_tk_2] = fcn(c0, alfa, tsim, pos_bar_vec, ksi_ld_hat_vec, tk_vec, pos_bar_tk_vec, ksi_ld_hat_tk_vec)
%%%% 更新事件触发时刻以及对应的状态反馈
iiuav = 2;
err_trig = pos_bar_vec(:,iiuav) - pos_bar_tk_vec(:,iiuav) - ( ksi_ld_hat_vec(:,iiuav) - ksi_ld_hat_tk_vec(:,iiuav) );
err_trig_norm = norm( err_trig(:), 2 );
err_trig_threshold = c0 * exp( -alfa * tsim );
if err_trig_norm >= err_trig_threshold
    tk_2 = tsim;
    pos_bar_tk_2 = pos_bar_vec(:,iiuav);
    ksi_ld_hat_tk_2 = ksi_ld_hat_vec(:,iiuav);
else
    tk_2 = tk_vec(iiuav);
    pos_bar_tk_2 = pos_bar_tk_vec(:,iiuav);
    ksi_ld_hat_tk_2 = ksi_ld_hat_tk_vec(:,iiuav);
end

== matlab function sim_tvt_2025_pos_ctrl/update event trigger state agent 3 ==
  data: tk_3 output; c0 input; alfa input; tsim input; pos_bar_vec input; ksi_ld_hat_vec input; tk_vec input; pos_bar_tk_vec input; pos_bar_tk_3 output; ksi_ld_hat_tk_3 output; ksi_ld_hat_tk_vec input
function [tk_3, pos_bar_tk_3, ksi_ld_hat_tk_3] = fcn(c0, alfa, tsim, pos_bar_vec, ksi_ld_hat_vec, tk_vec, pos_bar_tk_vec, ksi_ld_hat_tk_vec)
%%%% 更新事件触发时刻以及对应的状态反馈
iiuav = 3;
err_trig = pos_bar_vec(:,iiuav) - pos_bar_tk_vec(:,iiuav) - ( ksi_ld_hat_vec(:,iiuav) - ksi_ld_hat_tk_vec(:,iiuav) );
err_trig_norm = norm( err_trig(:), 2 );
err_trig_threshold = c0 * exp( -alfa * tsim );
if err_trig_norm >= err_trig_threshold
    tk_3 = tsim;
    pos_bar_tk_3 = pos_bar_vec(:,iiuav);
    ksi_ld_hat_tk_3 = ksi_ld_hat_vec(:,iiuav);
else
    tk_3 = tk_vec(iiuav);
    pos_bar_tk_3 = pos_bar_tk_vec(:,iiuav);
    ksi_ld_hat_tk_3 = ksi_ld_hat_tk_vec(:,iiuav);
end

== matlab function sim_tvt_2025_pos_ctrl/update event trigger state agent 4 ==
  data: tk_4 output; c0 input; alfa input; tsim input; pos_bar_vec input; ksi_ld_hat_vec input; tk_vec input; pos_bar_tk_vec input; pos_bar_tk_4 output; ksi_ld_hat_tk_4 output; ksi_ld_hat_tk_vec input
function [tk_4, pos_bar_tk_4, ksi_ld_hat_tk_4] = fcn(c0, alfa, tsim, pos_bar_vec, ksi_ld_hat_vec, tk_vec, pos_bar_tk_vec, ksi_ld_hat_tk_vec)
%%%% 更新事件触发时刻以及对应的状态反馈
iiuav = 4;
err_trig = pos_bar_vec(:,iiuav) - pos_bar_tk_vec(:,iiuav) - ( ksi_ld_hat_vec(:,iiuav) - ksi_ld_hat_tk_vec(:,iiuav) );
err_trig_norm = norm( err_trig(:), 2 );
err_trig_threshold = c0 * exp( -alfa * tsim );
if err_trig_norm >= err_trig_threshold
    tk_4 = tsim;
    pos_bar_tk_4 = pos_bar_vec(:,iiuav);
    ksi_ld_hat_tk_4 = ksi_ld_hat_vec(:,iiuav);
else
    tk_4 = tk_vec(iiuav);
    pos_bar_tk_4 = pos_bar_tk_vec(:,iiuav);
    ksi_ld_hat_tk_4 = ksi_ld_hat_tk_vec(:,iiuav);
end

== matlab function sim_tvt_2025_pos_ctrl/update event trigger state agent 5 ==
  data: tk_5 output; c0 input; alfa input; tsim input; pos_bar_vec input; ksi_ld_hat_vec input; tk_vec input; pos_bar_tk_vec input; pos_bar_tk_5 output; ksi_ld_hat_tk_5 output; ksi_ld_hat_tk_vec input
function [tk_5, pos_bar_tk_5, ksi_ld_hat_tk_5] = fcn(c0, alfa, tsim, pos_bar_vec, ksi_ld_hat_vec, tk_vec, pos_bar_tk_vec, ksi_ld_hat_tk_vec)
%%%% 更新事件触发时刻以及对应的状态反馈
iiuav = 5;
err_trig = pos_bar_vec(:,iiuav) - pos_bar_tk_vec(:,iiuav) - ( ksi_ld_hat_vec(:,iiuav) - ksi_ld_hat_tk_vec(:,iiuav) );
err_trig_norm = norm( err_trig(:), 2 );
err_trig_threshold = c0 * exp( -alfa * tsim );
if err_trig_norm >= err_trig_threshold
    tk_5 = tsim;
    pos_bar_tk_5 = pos_bar_vec(:,iiuav);
    ksi_ld_hat_tk_5 = ksi_ld_hat_vec(:,iiuav);
else
    tk_5 = tk_vec(iiuav);
    pos_bar_tk_5 = pos_bar_tk_vec(:,iiuav);
    ksi_ld_hat_tk_5 = ksi_ld_hat_tk_vec(:,iiuav);
end

== matlab function sim_tvt_2025_pos_ctrl/update betai agent 4 ==
  data: eps0 input; d_beta_hat_4 output; Wij input; Mii input; tsim input; u0 input; rho_hat_vec input
function d_beta_hat_4 = fcn(eps0, Wij, Mii, tsim, u0, rho_hat_vec)
%%%% 自适应律
iiuav = 4;
err_rho = Mii(iiuav, iiuav) * ( rho_hat_vec(:,iiuav) - u0(:) );
for jjuav = 1:5
    err_rho = err_rho + Wij(iiuav, jjuav) * ( rho_hat_vec(:,iiuav) - rho_hat_vec(:,jjuav) );
end
d_beta_hat_4 = ( err_rho(:)' ) * tanh( err_rho(:) ./ exp( -eps0 * tsim ) );

== matlab function sim_tvt_2025_pos_ctrl/combine event trigger tk ==
  data: tk_1 input; tk_vec output; tk_2 input; tk_3 input; tk_4 input; tk_5 input
function tk_vec  = fcn(tk_1, tk_2, tk_3, tk_4, tk_5)
%%%% 合并事件触发时间
tk_vec  = [tk_1, tk_2, tk_3, tk_4, tk_5];

== matlab function sim_tvt_2025_pos_ctrl/combine event trigger pos_bar_tk ==
  data: pos_bar_tk_1 input; pos_bar_tk_vec output; pos_bar_tk_2 input; pos_bar_tk_3 input; pos_bar_tk_4 input; pos_bar_tk_5 input
function pos_bar_tk_vec  = fcn(pos_bar_tk_1, pos_bar_tk_2, pos_bar_tk_3, pos_bar_tk_4, pos_bar_tk_5)
%%%% 合并事件触发的辅助位置向量状态反馈
pos_bar_tk_vec  = zeros(3,5);
pos_bar_tk_vec(:,1) = pos_bar_tk_1(:);
pos_bar_tk_vec(:,2) = pos_bar_tk_2(:);
pos_bar_tk_vec(:,3) = pos_bar_tk_3(:);
pos_bar_tk_vec(:,4) = pos_bar_tk_4(:);
pos_bar_tk_vec(:,5) = pos_bar_tk_5(:);

== matlab function sim_tvt_2025_pos_ctrl/combine event trigger ksi_ld_hat_tk ==
  data: ksi_ld_hat_tk_1 input; ksi_ld_hat_tk_vec output; ksi_ld_hat_tk_2 input; ksi_ld_hat_tk_3 input; ksi_ld_hat_tk_4 input; ksi_ld_hat_tk_5 input
function ksi_ld_hat_tk_vec  = fcn(ksi_ld_hat_tk_1, ksi_ld_hat_tk_2, ksi_ld_hat_tk_3, ksi_ld_hat_tk_4, ksi_ld_hat_tk_5)
%%%% 合并事件触发的领导者位置估计状态反馈
ksi_ld_hat_tk_vec  = zeros(3,5);
ksi_ld_hat_tk_vec(:,1) = ksi_ld_hat_tk_1(:);
ksi_ld_hat_tk_vec(:,2) = ksi_ld_hat_tk_2(:);
ksi_ld_hat_tk_vec(:,3) = ksi_ld_hat_tk_3(:);
ksi_ld_hat_tk_vec(:,4) = ksi_ld_hat_tk_4(:);
ksi_ld_hat_tk_vec(:,5) = ksi_ld_hat_tk_5(:);

== matlab function sim_tvt_2025_pos_ctrl/cal Di agent 1 ==
  data: Di_1 output; Wij input; delta_ksi_vec input; pos_bar_tk_vec input; ksi_ld_hat_tk_vec input; ksi_ld_hat_vec input
function Di_1 = fcn(Wij, delta_ksi_vec, pos_bar_tk_vec, ksi_ld_hat_tk_vec, ksi_ld_hat_vec)
%%%% 更新事件触发分布式误差
iiuav = 1;
Di_1 = zeros(3,1);
for jjuav = 1:5
    Di_1 = Di_1 + Wij(iiuav,jjuav) * ( pos_bar_tk_vec(:,jjuav) ...
                    + ( ksi_ld_hat_vec(:,jjuav) - ksi_ld_hat_tk_vec(:,jjuav) ) ...
                    + ( delta_ksi_vec(:,iiuav) - delta_ksi_vec(:,jjuav) ) );
end

== matlab function sim_tvt_2025_pos_ctrl/cal Di agent 2 ==
  data: Di_2 output; Wij input; delta_ksi_vec input; pos_bar_tk_vec input; ksi_ld_hat_tk_vec input; ksi_ld_hat_vec input
function Di_2 = fcn(Wij, delta_ksi_vec, pos_bar_tk_vec, ksi_ld_hat_tk_vec, ksi_ld_hat_vec)
%%%% 更新事件触发分布式误差
iiuav = 2;
Di_2 = zeros(3,1);
for jjuav = 1:5
    Di_2 = Di_2 + Wij(iiuav,jjuav) * ( pos_bar_tk_vec(:,jjuav) ...
                    + ( ksi_ld_hat_vec(:,jjuav) - ksi_ld_hat_tk_vec(:,jjuav) ) ...
                    + ( delta_ksi_vec(:,iiuav) - delta_ksi_vec(:,jjuav) ) );
end

== matlab function sim_tvt_2025_pos_ctrl/cal Di agent 3 ==
  data: Di_3 output; Wij input; delta_ksi_vec input; pos_bar_tk_vec input; ksi_ld_hat_tk_vec input; ksi_ld_hat_vec input
function Di_3 = fcn(Wij, delta_ksi_vec, pos_bar_tk_vec, ksi_ld_hat_tk_vec, ksi_ld_hat_vec)
%%%% 更新事件触发分布式误差
iiuav = 3;
Di_3 = zeros(3,1);
for jjuav = 1:5
    Di_3 = Di_3 + Wij(iiuav,jjuav) * ( pos_bar_tk_vec(:,jjuav) ...
                    + ( ksi_ld_hat_vec(:,jjuav) - ksi_ld_hat_tk_vec(:,jjuav) ) ...
                    + ( delta_ksi_vec(:,iiuav) - delta_ksi_vec(:,jjuav) ) );
end

== matlab function sim_tvt_2025_pos_ctrl/cal Di agent 4 ==
  data: Di_4 output; Wij input; delta_ksi_vec input; pos_bar_tk_vec input; ksi_ld_hat_tk_vec input; ksi_ld_hat_vec input
function Di_4 = fcn(Wij, delta_ksi_vec, pos_bar_tk_vec, ksi_ld_hat_tk_vec, ksi_ld_hat_vec)
%%%% 更新事件触发分布式误差
iiuav = 4;
Di_4 = zeros(3,1);
for jjuav = 1:5
    Di_4 = Di_4 + Wij(iiuav,jjuav) * ( pos_bar_tk_vec(:,jjuav) ...
                    + ( ksi_ld_hat_vec(:,jjuav) - ksi_ld_hat_tk_vec(:,jjuav) ) ...
                    + ( delta_ksi_vec(:,iiuav) - delta_ksi_vec(:,jjuav) ) );
end

== matlab function sim_tvt_2025_pos_ctrl/cal Di agent 5 ==
  data: Di_5 output; Wij input; delta_ksi_vec input; pos_bar_tk_vec input; ksi_ld_hat_tk_vec input; ksi_ld_hat_vec input
function Di_5 = fcn(Wij, delta_ksi_vec, pos_bar_tk_vec, ksi_ld_hat_tk_vec, ksi_ld_hat_vec)
%%%% 更新事件触发分布式误差
iiuav = 5;
Di_5 = zeros(3,1);
for jjuav = 1:5
    Di_5 = Di_5 + Wij(iiuav,jjuav) * ( pos_bar_tk_vec(:,jjuav) ...
                    + ( ksi_ld_hat_vec(:,jjuav) - ksi_ld_hat_tk_vec(:,jjuav) ) ...
                    + ( delta_ksi_vec(:,iiuav) - delta_ksi_vec(:,jjuav) ) );
end

== matlab function sim_tvt_2025_pos_ctrl/combine Di_vec ==
  data: Di_1 input; Di_vec output; Di_2 input; Di_3 input; Di_4 input; Di_5 input
function Di_vec  = fcn(Di_1, Di_2, Di_3, Di_4, Di_5)
%%%% 合并辅助位置向量
Di_vec = zeros(3,5);
Di_vec(:,1) = Di_1(:);
Di_vec(:,2) = Di_2(:);
Di_vec(:,3) = Di_3(:);
Di_vec(:,4) = Di_4(:);
Di_vec(:,5) = Di_5(:);

== matlab function sim_tvt_2025_pos_ctrl/cal x4i agent 1 ==
  data: d_x4i_1 output; Wij input; lam4 input; x4i_vec input; Di_vec input; eta_ld_hat_vec input
function d_x4i_1 = fcn(Wij, lam4, x4i_vec, Di_vec, eta_ld_hat_vec)
%%%% 更新高阶系统的四阶状态量
iiuav = 1;
d_x4i_1 = lam4 * Di_vec(:,iiuav) + eta_ld_hat_vec(:,iiuav);
for jjuav = 1:5
    d_x4i_1 = d_x4i_1 - lam4 * Wij(iiuav,jjuav) * x4i_vec(:,iiuav);
end

== matlab function sim_tvt_2025_pos_ctrl/cal x4i agent 2 ==
  data: d_x4i_2 output; Wij input; lam4 input; x4i_vec input; Di_vec input; eta_ld_hat_vec input
function d_x4i_2 = fcn(Wij, lam4, x4i_vec, Di_vec, eta_ld_hat_vec)
%%%% 更新高阶系统的四阶状态量
iiuav = 2;
d_x4i_2 = lam4 * Di_vec(:,iiuav) + eta_ld_hat_vec(:,iiuav);
for jjuav = 1:5
    d_x4i_2 = d_x4i_2 - lam4 * Wij(iiuav,jjuav) * x4i_vec(:,iiuav);
end

== matlab function sim_tvt_2025_pos_ctrl/update betai agent 5 ==
  data: eps0 input; d_beta_hat_5 output; Wij input; Mii input; tsim input; u0 input; rho_hat_vec input
function d_beta_hat_5 = fcn(eps0, Wij, Mii, tsim, u0, rho_hat_vec)
%%%% 自适应律
iiuav = 5;
err_rho = Mii(iiuav, iiuav) * ( rho_hat_vec(:,iiuav) - u0(:) );
for jjuav = 1:5
    err_rho = err_rho + Wij(iiuav, jjuav) * ( rho_hat_vec(:,iiuav) - rho_hat_vec(:,jjuav) );
end
d_beta_hat_5 = ( err_rho(:)' ) * tanh( err_rho(:) ./ exp( -eps0 * tsim ) );

== matlab function sim_tvt_2025_pos_ctrl/cal x4i agent 3 ==
  data: d_x4i_3 output; Wij input; lam4 input; x4i_vec input; Di_vec input; eta_ld_hat_vec input
function d_x4i_3 = fcn(Wij, lam4, x4i_vec, Di_vec, eta_ld_hat_vec)
%%%% 更新高阶系统的四阶状态量
iiuav = 3;
d_x4i_3 = lam4 * Di_vec(:,iiuav) + eta_ld_hat_vec(:,iiuav);
for jjuav = 1:5
    d_x4i_3 = d_x4i_3 - lam4 * Wij(iiuav,jjuav) * x4i_vec(:,iiuav);
end

== matlab function sim_tvt_2025_pos_ctrl/cal x4i agent 4 ==
  data: d_x4i_4 output; Wij input; lam4 input; x4i_vec input; Di_vec input; eta_ld_hat_vec input
function d_x4i_4 = fcn(Wij, lam4, x4i_vec, Di_vec, eta_ld_hat_vec)
%%%% 更新高阶系统的四阶状态量
iiuav = 4;
d_x4i_4 = lam4 * Di_vec(:,iiuav) + eta_ld_hat_vec(:,iiuav);
for jjuav = 1:5
    d_x4i_4 = d_x4i_4 - lam4 * Wij(iiuav,jjuav) * x4i_vec(:,iiuav);
end

== matlab function sim_tvt_2025_pos_ctrl/cal x4i agent 5 ==
  data: d_x4i_5 output; Wij input; lam4 input; x4i_vec input; Di_vec input; eta_ld_hat_vec input
function d_x4i_5 = fcn(Wij, lam4, x4i_vec, Di_vec, eta_ld_hat_vec)
%%%% 更新高阶系统的四阶状态量
iiuav = 5;
d_x4i_5 = lam4 * Di_vec(:,iiuav) + eta_ld_hat_vec(:,iiuav);
for jjuav = 1:5
    d_x4i_5 = d_x4i_5 - lam4 * Wij(iiuav,jjuav) * x4i_vec(:,iiuav);
end

== matlab function sim_tvt_2025_pos_ctrl/combine x4i ==
  data: x4i_1 input; x4i_vec output; x4i_2 input; x4i_3 input; x4i_4 input; x4i_5 input
function x4i_vec  = fcn(x4i_1, x4i_2, x4i_3, x4i_4, x4i_5)
%%%% 合并高阶系统的四阶状态量
x4i_vec = zeros(3,5);
x4i_vec(:,1) = x4i_1(:);
x4i_vec(:,2) = x4i_2(:);
x4i_vec(:,3) = x4i_3(:);
x4i_vec(:,4) = x4i_4(:);
x4i_vec(:,5) = x4i_5(:);

== matlab function sim_tvt_2025_pos_ctrl/cal x3i agent 1 ==
  data: d_x3i_1 output; lam3 input; x3i_vec input; x4i_vec input; eta_ld_hat_vec input
function d_x3i_1 = fcn(lam3, x3i_vec, x4i_vec, eta_ld_hat_vec)
%%%% 更新高阶系统的三阶状态量
iiuav = 1;
d_x3i_1 = lam3 * ( x4i_vec(:,iiuav) - x3i_vec(:,iiuav) ) + eta_ld_hat_vec(:,iiuav);

== matlab function sim_tvt_2025_pos_ctrl/cal x3i agent 2 ==
  data: d_x3i_2 output; lam3 input; x3i_vec input; x4i_vec input; eta_ld_hat_vec input
function d_x3i_2 = fcn(lam3, x3i_vec, x4i_vec, eta_ld_hat_vec)
%%%% 更新高阶系统的三阶状态量
iiuav = 2;
d_x3i_2 = lam3 * ( x4i_vec(:,iiuav) - x3i_vec(:,iiuav) ) + eta_ld_hat_vec(:,iiuav);

== matlab function sim_tvt_2025_pos_ctrl/cal x3i agent 3 ==
  data: d_x3i_3 output; lam3 input; x3i_vec input; x4i_vec input; eta_ld_hat_vec input
function d_x3i_3 = fcn(lam3, x3i_vec, x4i_vec, eta_ld_hat_vec)
%%%% 更新高阶系统的三阶状态量
iiuav = 3;
d_x3i_3 = lam3 * ( x4i_vec(:,iiuav) - x3i_vec(:,iiuav) ) + eta_ld_hat_vec(:,iiuav);

== matlab function sim_tvt_2025_pos_ctrl/cal x3i agent 4 ==
  data: d_x3i_4 output; lam3 input; x3i_vec input; x4i_vec input; eta_ld_hat_vec input
function d_x3i_4 = fcn(lam3, x3i_vec, x4i_vec, eta_ld_hat_vec)
%%%% 更新高阶系统的三阶状态量
iiuav = 4;
d_x3i_4 = lam3 * ( x4i_vec(:,iiuav) - x3i_vec(:,iiuav) ) + eta_ld_hat_vec(:,iiuav);

== matlab function sim_tvt_2025_pos_ctrl/cal x3i agent 5 ==
  data: d_x3i_5 output; lam3 input; x3i_vec input; x4i_vec input; eta_ld_hat_vec input
function d_x3i_5 = fcn(lam3, x3i_vec, x4i_vec, eta_ld_hat_vec)
%%%% 更新高阶系统的三阶状态量
iiuav = 5;
d_x3i_5 = lam3 * ( x4i_vec(:,iiuav) - x3i_vec(:,iiuav) ) + eta_ld_hat_vec(:,iiuav);

== matlab function sim_tvt_2025_pos_ctrl/combine x3i ==
  data: x3i_1 input; x3i_vec output; x3i_2 input; x3i_3 input; x3i_4 input; x3i_5 input
function x3i_vec  = fcn(x3i_1, x3i_2, x3i_3, x3i_4, x3i_5)
%%%% 合并高阶系统的三阶状态量
x3i_vec = zeros(3,5);
x3i_vec(:,1) = x3i_1(:);
x3i_vec(:,2) = x3i_2(:);
x3i_vec(:,3) = x3i_3(:);
x3i_vec(:,4) = x3i_4(:);
x3i_vec(:,5) = x3i_5(:);

== matlab function sim_tvt_2025_pos_ctrl/cal x2i agent 1 ==
  data: d_x2i_1 output; lam2 input; x2i_vec input; x3i_vec input; eta_ld_hat_vec input
function d_x2i_1 = fcn(lam2, x2i_vec, x3i_vec, eta_ld_hat_vec)
%%%% 更新高阶系统的二阶状态量
iiuav = 1;
d_x2i_1 = lam2 * ( x3i_vec(:,iiuav) - x2i_vec(:,iiuav) ) + eta_ld_hat_vec(:,iiuav);

== matlab function sim_tvt_2025_pos_ctrl/combine betai1 ==
  data: sigmai_1 input; sigmai_vec output; sigmai_2 input; sigmai_3 input; sigmai_4 input; sigmai_5 input
function sigmai_vec  = fcn(sigmai_1, sigmai_2, sigmai_3, sigmai_4, sigmai_5)
%%%% 合并分布式观测器变量
sigmai_vec = zeros(3,5);
sigmai_vec(:,1) = sigmai_1(:);
sigmai_vec(:,2) = sigmai_2(:);
sigmai_vec(:,3) = sigmai_3(:);
sigmai_vec(:,4) = sigmai_4(:);
sigmai_vec(:,5) = sigmai_5(:);

== matlab function sim_tvt_2025_pos_ctrl/cal x2i agent 2 ==
  data: d_x2i_2 output; lam2 input; x2i_vec input; x3i_vec input; eta_ld_hat_vec input
function d_x2i_2 = fcn(lam2, x2i_vec, x3i_vec, eta_ld_hat_vec)
%%%% 更新高阶系统的二阶状态量
iiuav = 2;
d_x2i_2 = lam2 * ( x3i_vec(:,iiuav) - x2i_vec(:,iiuav) ) + eta_ld_hat_vec(:,iiuav);
